simulink model "vehiclemodel"  (R2021b)
settings: Solver=VariableStepAuto  StartTime=0.0  StopTime=300  RelTol=1e-3
libraries: vehdynlibsteering x1, autolibshared x1
settings Model: Creator=alokpunjbagrodia  LastModifiedBy=alokpunjbagrodia

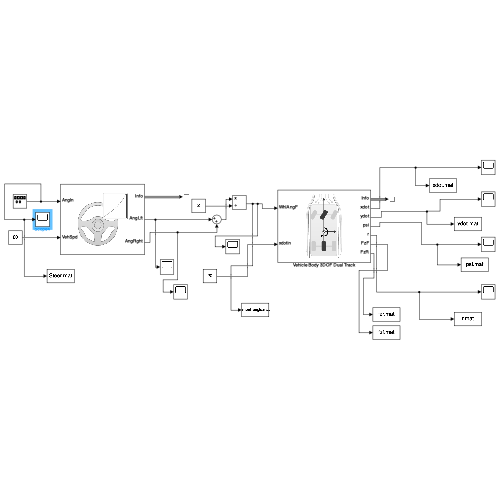
[thumbnail: Simulink's stored preview of the top-level diagram]
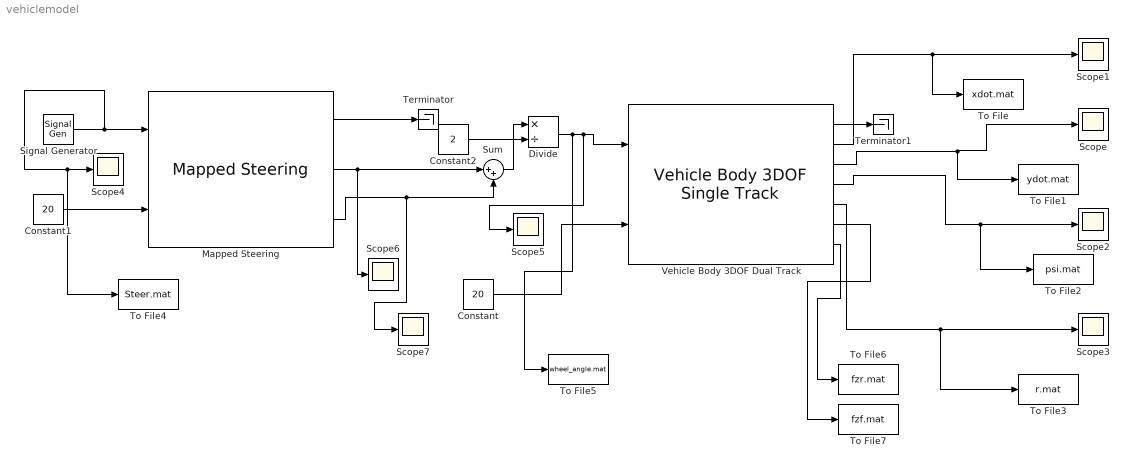
== system vehiclemodel ==
  Constant : Constant  Value=20  SampleTime=0.01
  Constant1 : Constant  Value=20  SampleTime=0.01
  Constant2 : Constant  Value=2  SampleTime=0.01
  Divide : Product  Inputs=*/
  Mapped Steering : vehdynlibsteering/Mapped Steering  SpdDpd=on  StrgAngBpts=[-1.5*pi 1.5*pi]  WhlLftTbl=[-1.5*pi 1.5*pi]/13.5  WhlRghtTbl=[-1.5*pi 1.5*pi]/13.5  VehSpdBpts=[-1 1]  SpdFctTbl=[1 1]  aMode=2
      settings: SourceProductBaseCode=VE
  Scope{,1..7} (8 alike) : Scope
  Signal Generator : SignalGenerator  Amplitude=0.1  Frequency=0.09  Units=rad/sec
  Sum : Sum  Inputs=|++
  Terminator : Terminator
  Terminator1 : Terminator
  To File : ToFile  Filename=xdot.mat  MatrixName=xdot  SampleTime=0.01
  To File1 : ToFile  Filename=ydot.mat  MatrixName=ydot  SampleTime=0.01
  To File2 : ToFile  Filename=psi.mat  MatrixName=psi  SampleTime=0.01
  To File3 : ToFile  Filename=r.mat  MatrixName=r  SampleTime=0.01
  To File4 : ToFile  Filename=Steer.mat  SampleTime=0.01
  To File5 : ToFile  Filename=wheel_angle.mat  MatrixName=wheel_angle  SampleTime=0.01
  To File6 : ToFile  Filename=fzr.mat  MatrixName=fzr  SampleTime=0.01
  To File7 : ToFile  Filename=fzf.mat  MatrixName=fzf  SampleTime=0.01
  Vehicle Body 3DOF Dual Track : autolibshared/Vehicle Body 3DOF Single Track  trackMode=Single (bicycle)  inputMode=External longitudinal velocity  frontSteerMode=on  rearSteerMode=off  windMode=off  muMode=off  extFMode=off  extMMode=off  htchFMode=off  htchMMode=off  extXo=off  extpsio=off  extxdoto=off  extro=off  extYo=off  extTamb=off  extydoto=off  aMode=2  NF=2  NR=2  m=2000  a=1.4  b=1.6  h=0.35  dh=1  hh=0.2  X_o=0  xdot_o=0  CalphaMode=off  sigmaMode=on  d=0  hl=0  w=[1.4,1.4]  Cy_f=12e3  Cy_r=11e3  sigma_f=.1  sigma_r=.1  alpha_f_brk=[-.1 .1]  Cy_f_data=[-9e3 9e3]  alpha_r_brk=[-.1 .1]  Cy_r_data=[-9e3 9e3]  Y_o=0  ydot_o=0  Izz=4000  psi_o=0  r_o=0  Af=2  Cd=.3  Cl=.1  Cpm=.1  beta_w=[0 0.01:0.01:0.3]  Cs=[0 0.01:0.01:0.3]  Cym=[0 1e-6:0.01:0.3]  Pabs=101325  Tair=273  g=9.81  mu=1  xdot_tol=.01  Fznom=5000  Fxtire_sat=7e4  Fytire_sat=7e4  longOff=0  latOff=0  vertOff=0  wrapAng=off
      settings: SourceProductBaseCode=PW,DR,MT,UV,VE
  wires:
  Signal Generator/1 -> To File4/1, Scope4/1, Mapped Steering/1
  Constant/1 -> Vehicle Body 3DOF Dual Track/2
  Vehicle Body 3DOF Dual Track/1 -> Terminator1/1
  Vehicle Body 3DOF Dual Track/3 -> To File1/1, Scope/1
  Vehicle Body 3DOF Dual Track/2 -> To File/1, Scope1/1
  Vehicle Body 3DOF Dual Track/4 -> To File2/1, Scope2/1
  Vehicle Body 3DOF Dual Track/5 -> To File3/1, Scope3/1
  Vehicle Body 3DOF Dual Track/6 -> To File7/1
  Vehicle Body 3DOF Dual Track/7 -> To File6/1
  Constant1/1 -> Mapped Steering/2
  Mapped Steering/1 -> Terminator/1
  Mapped Steering/2 -> Sum/1, Scope6/1
  Mapped Steering/3 -> Sum/2, Scope7/1
  Sum/1 -> Divide/1
  Constant2/1 -> Divide/2
  Divide/1 -> To File5/1, Scope5/1, Vehicle Body 3DOF Dual Track/1
